simulink model "A5_IMC_control"  (R2023a)
settings: Solver=VariableStepAuto  StartTime=0.0  StopTime=20  RelTol=1e-3
values from neighbouring files (symbols this model uses):
  CA0 = 0.9803    [A2_Task9_param_consts.m]
  CAf = 1.0    (= 1)    [A1_find_steady_state.m]    (also in A2_Task9_param_consts.m)
  Cp = 0.239    [A1_find_steady_state.m]    (also in A2_Task9_param_consts.m)
  dHr = -5e4    (= -50000)    [A1_find_steady_state.m]    (also in A2_Task9_param_consts.m)
  ER = 8750    [A1_find_steady_state.m]    (also in A2_Task9_param_consts.m)
  k0 = 6.379829e10    (= 63798290000)    [A1_find_steady_state.m]    (also in A2_Task9_param_consts.m)
  Km = 0.858176    [A2_Task9_param_consts.m]    (also in A4_task9_fopdt.m = dy / du)
  q = 100    [A1_find_steady_state.m]    (also in A2_Task9_param_consts.m)
  rho = 1000    [A1_find_steady_state.m]    (also in A2_Task9_param_consts.m)
  T0 = 303.49    [A2_Task9_param_consts.m]
  tau_f = 0.41534    [A2_Task9_param_consts.m]
  taum = 0.41534    [A2_Task9_param_consts.m]
  Tf = 350    [A1_find_steady_state.m]    (also in A2_Task9_param_consts.m)
  UA = 5e4    (= 50000)    [A1_find_steady_state.m]    (also in A2_Task9_param_consts.m)
  V = 100    [A1_find_steady_state.m]    (also in A2_Task9_param_consts.m)
settings Model: Creator=xiong  LastModifiedBy=xiong

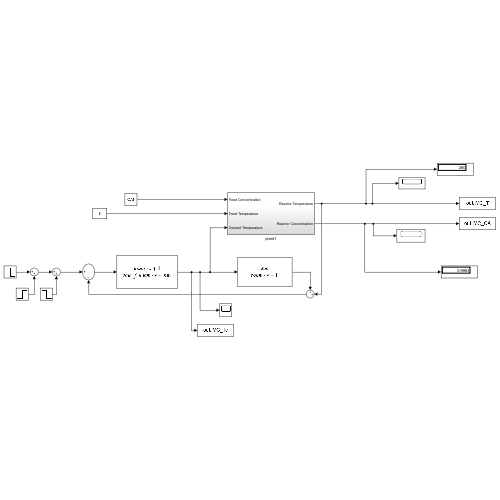
[thumbnail: Simulink's stored preview of the top-level diagram]
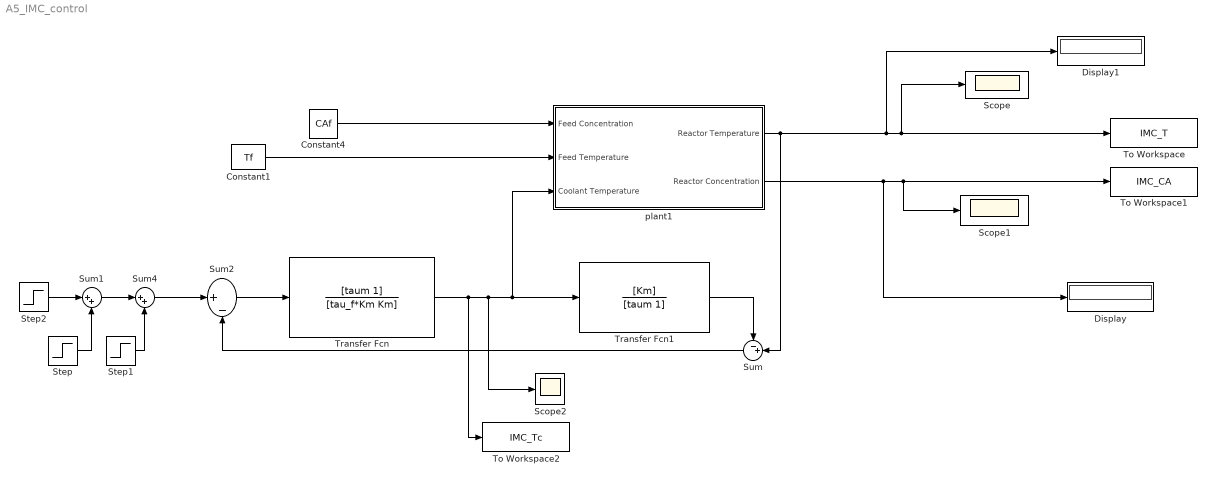
== system A5_IMC_control ==
  Constant1 : Constant  Value=Tf
  Constant4 : Constant  Value=CAf
  Display : Display
  Display1 : Display
  Scope : Scope
  Scope1 : Scope
  Scope2 : Scope
  Step : Step  Time=8  After=20  SampleTime=0.1
  Step1 : Step  Time=12  After=-40  SampleTime=0.1
  Step2 : Step  Time=4  Before=303  After=300  SampleTime=0.1
  Sum : Sum  Inputs=-+|
  Sum1 : Sum  Inputs=|++
  Sum2 : Sum  Inputs=|+-
  Sum4 : Sum  Inputs=|++
  To Workspace : ToWorkspace  VariableName=IMC_T  SaveFormat=Timeseries  SampleTime=-1
  To Workspace1 : ToWorkspace  VariableName=IMC_CA  SaveFormat=Timeseries  SampleTime=-1
  To Workspace2 : ToWorkspace  VariableName=IMC_Tc  SaveFormat=Timeseries  SampleTime=-1
  Transfer Fcn : TransferFcn  Numerator=[taum 1]  Denominator=[tau_f*Km Km]
  Transfer Fcn1 : TransferFcn  Numerator=[Km]  Denominator=[taum 1]
  plant1 : Subsystem
  wires:
  plant1/1(Reactor Temperature) -> Display1/1, To Workspace/1, Scope/1, Sum/2
  Step2/1 -> Sum1/1
  plant1/2(Reactor Concentration) -> To Workspace1/1, Scope1/1, Display/1
  Sum2/1 -> Transfer Fcn/1
  Constant4/1 -> plant1/1(Feed Concentration)
  Constant1/1 -> plant1/2(Feed Temperature)
  Transfer Fcn1/1 -> Sum/1
  Transfer Fcn/1 -> plant1/3(Coolant Temperature), Transfer Fcn1/1, Scope2/1, To Workspace2/1
  Sum1/1 -> Sum4/1
  Step/1 -> Sum1/2
  Step1/1 -> Sum4/2
  Sum4/1 -> Sum2/1
  Sum/1 -> Sum2/2

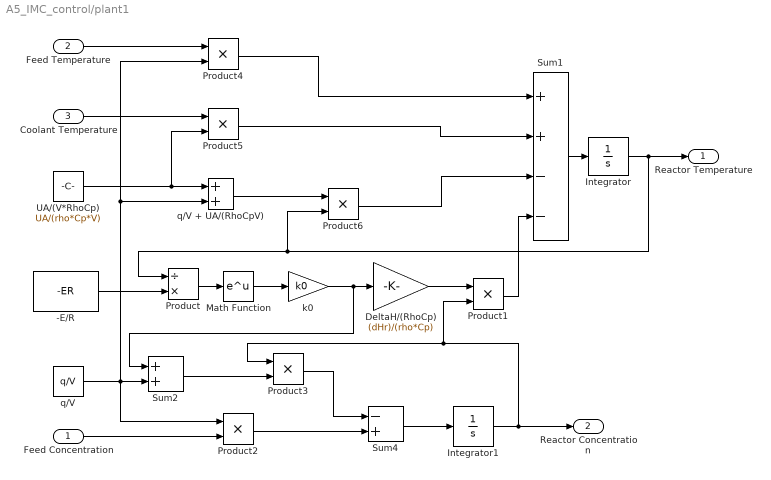
== system A5_IMC_control/plant1 ==
  Feed Concentration : Inport
  Feed Temperature : Inport  Port=2
  Coolant Temperature : Inport  Port=3
  -E/R : Constant  Value=-ER
  DeltaH/(RhoCp) : Gain  Gain=(dHr)/(rho*Cp)  SaturateOnIntegerOverflow=on  OutDataTypeStr=Inherit: Same as input  ParamDataTypeStr=Inherit: Same as input
  Integrator : Integrator  InitialCondition=T0  LimitOutput=on  LowerSaturationLimit=0
  Integrator1 : Integrator  InitialCondition=CA0  LimitOutput=on  LowerSaturationLimit=0
  Math Function : Math  SignedPower=on
  Product : Product  Inputs=/*  InputSameDT=on  RndMeth=Zero  SaturateOnIntegerOverflow=on  OutDataTypeStr=Inherit: Same as first input
  Product1 : Product  InputSameDT=on  RndMeth=Zero  SaturateOnIntegerOverflow=on  OutDataTypeStr=Inherit: Same as first input
  Product{2,4..6} (4 alike) : Product
  Product3 : Product  InputSameDT=on  RndMeth=Zero  SaturateOnIntegerOverflow=on  OutDataTypeStr=Inherit: Same as first input
  Sum1 : Sum  Inputs=++--  InputSameDT=on  SaturateOnIntegerOverflow=on  OutDataTypeStr=Inherit: Same as first input
  Sum2 : Sum  InputSameDT=on  SaturateOnIntegerOverflow=on  OutDataTypeStr=Inherit: Same as first input
  Sum4 : Sum  Inputs=-+  InputSameDT=on  SaturateOnIntegerOverflow=on  OutDataTypeStr=Inherit: Same as first input
  UA/(V*RhoCp) : Constant  Value=UA/(rho*Cp*V)
  k0 : Gain  Gain=k0  SaturateOnIntegerOverflow=on  OutDataTypeStr=Inherit: Same as input  ParamDataTypeStr=Inherit: Same as input
  q/V : Constant  Value=q/V
  q/V + UA/(RhoCpV) : Sum
  Reactor Temperature : Outport
  Reactor Concentration : Outport  Port=2
  wires:
  Product4/1 -> Sum1/1
  Sum1/1 -> Integrator/1
  Integrator/1 -> Product6/2, Product/1, Reactor Temperature/1
  Product5/1 -> Sum1/2
  Product6/1 -> Sum1/3
  Product/1 -> Math Function/1
  Math Function/1 -> k0/1
  DeltaH/(RhoCp)/1 -> Product1/1
  Product1/1 -> Sum1/4
  k0/1 -> DeltaH/(RhoCp)/1, Sum2/1
  -E/R/1 -> Product/2
  Product3/1 -> Sum4/1
  Sum4/1 -> Integrator1/1
  Integrator1/1 -> Product1/2, Product3/1, Reactor Concentration/1
  q/V/1 -> Product2/1, Sum2/2, Product4/2, q/V + UA/(RhoCpV)/2
  Product2/1 -> Sum4/2
  Feed Temperature/1 -> Product4/1
  Feed Concentration/1 -> Product2/2
  Coolant Temperature/1 -> Product5/1
  Sum2/1 -> Product3/2
  UA/(V*RhoCp)/1 -> Product5/2, q/V + UA/(RhoCpV)/1
  q/V + UA/(RhoCpV)/1 -> Product6/1
